simulink model "C02_PID_tuning_SISO"  (R2016b)
settings: Solver=ode45  StartTime=0.0  StopTime=4.5  RelTol=1e-3  EnableMultiTasking=on
model workspace (MAT data in the model file):
  sintez_sys_stab_optim : sldodialogs.data.SessionData (value not decoded)
undefined symbols (not defined in the file or in its folder): Kd, Ki, Kp
libraries: checkpacklib x1
settings Model: Creator=Gamno  LastModifiedBy=Maksim
settings DataIOCC: LimitDataPoints=on  SaveFormat=Array
settings OptimizationCC: ExpressionDepthLimit=2147483647  LifeSpan=inf
settings DebuggingCC: UnderspecifiedInitializationDetection=Classic  MergeDetectMultiDrivingBlocksExec=none  SolverPrmCheckMsg=warning  FcnCallInpInsideContextMsg=warning  StateNameClashWarn=warning  SFUnexpectedBacktrackingDiag=warning  SFNoUnconditionalDefaultTransitionDiag=warning  SFExecutionAtInitializationDiag=none
settings HardwareCC: ProdBitPerPointer=32  ProdBitPerSizeT=32  ProdBitPerPtrDiffT=32  ProdLargestAtomicFloat=None  ProdIntDivRoundTo=Undefined  ProdEndianess=Unspecified  ProdWordSize=32  ProdHWDeviceType=32-bit Generic
settings ModelReferenceCC: PropagateSignalLabelsOutOfModel=off
settings GRTTargetCC: TargetLangStandard=C89/C90 (ANSI)  GeneratePreprocessorConditionals=Disable all  CombineOutputUpdateFcns=off  GRTInterface=on
settings ConfigComp: CovMetricSettings=dw  CovHtmlReporting=on  CovSaveCumulativeToWorkspaceVar=on  CovSaveSingleToWorkspaceVar=on  CovExternalEMLEnable=off

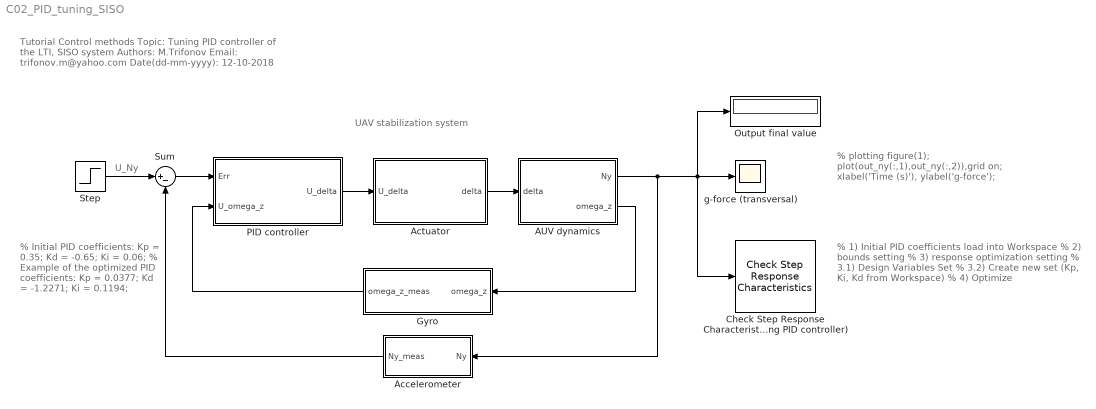
== system C02_PID_tuning_SISO ==
  note: UAV stabilization system
  note: % Initial PID coefficients:
      | Kp = 0.35;
      | Kd = -0.65;
      | Ki = 0.06;
      |
      | % Example of the optimized
      | PID coefficients:
      | Kp = 0.0377;
      | Kd = -1.2271;
      | Ki = 0.1194;
  note: U_Ny
  note: Tutorial Control methods
      | Topic: Tuning PID controller of the LTI, SISO system
      | Authors: M.Trifonov
      | Email: trifonov.m@yahoo.com
      | Date(dd-mm-yyyy): 12-10-2018
  note: % plotting
      | figure(1);
      | plot(out_ny(:,1),out_ny(:,2)),grid on;
      | xlabel('Time (s)'), ylabel('g-force');
  note: % 1) Initial PID coefficients load into Workspace
      | % 2) bounds setting
      | % 3) response optimization setting
      | % 3.1) Design Variables Set
      | % 3.2) Create new set (Kp, Ki, Kd from Workspace)
      | % 4) Optimize
  AUV dynamics : Subsystem
  Accelerometer : Subsystem
  Actuator : Subsystem
  Check Step Response Characteristics (tuning PID controller) : checkpacklib/Check Step Response  Characteristics  InstantiateOnLoad=on  enabled=on  stopWhenAssertionFail=off  export=off  ViewDlgPos=[1 41 1366 651]  OpenViewOnLoad=off  LaunchViewOnOpen=off  TimeUnits=seconds  EnableStepResponseBound=on  InitialValue=0  FinalValue=20  StepTime=0  RiseTime=1  PercentRise=90  SettlingTime=3  PercentSettling=1  PercentOvershoot=20  PercentUndershoot=1
  Gyro : Subsystem
  Output final value : Display
  PID controller : Subsystem
  Step : Step  Time=0  After=20  SampleTime=0
  Sum : Sum  Inputs=|+-
  g-force (transversal) : Scope
  wires:
  Step/1 -> Sum/1
  AUV dynamics/1(Ny) -> Output final value/1, Check Step Response Characteristics (tuning PID controller)/1, g-force (transversal)/1, Accelerometer/1(Ny)
  Sum/1 -> PID controller/1(Err)
  PID controller/1(U_delta) -> Actuator/1(U_delta)
  Actuator/1(delta) -> AUV dynamics/1(delta)
  AUV dynamics/2(omega_z) -> Gyro/1(omega_z)
  Gyro/1(omega_z_meas) -> PID controller/2(U_omega_z)
  Accelerometer/1(Ny_meas) -> Sum/2

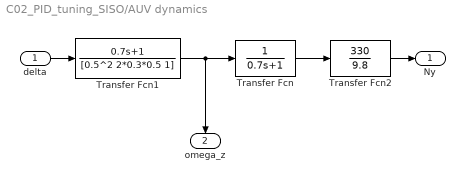
== system C02_PID_tuning_SISO/AUV dynamics ==
  delta : Inport
  Transfer Fcn : TransferFcn  Denominator=[0.7 1]
  Transfer Fcn1 : TransferFcn  Numerator=[0.7 1]  Denominator=[0.5^2 2*0.3*0.5 1]
  Transfer Fcn2 : TransferFcn  Numerator=[330]  Denominator=[9.8]
  Ny : Outport
  omega_z : Outport  Port=2
  wires:
  Transfer Fcn/1 -> Transfer Fcn2/1
  Transfer Fcn1/1 -> Transfer Fcn/1, omega_z/1
  delta/1 -> Transfer Fcn1/1
  Transfer Fcn2/1 -> Ny/1

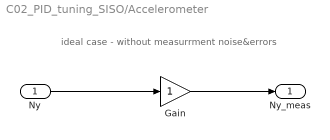
== system C02_PID_tuning_SISO/Accelerometer ==
  note: ideal case - without measurrment noise&errors
  Ny : Inport
  Gain : Gain
  Ny_meas : Outport
  wires:
  Gain/1 -> Ny_meas/1
  Ny/1 -> Gain/1

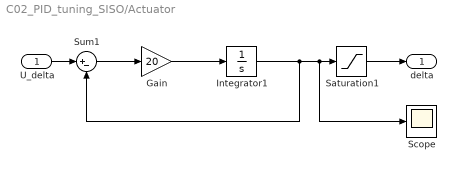
== system C02_PID_tuning_SISO/Actuator ==
  U_delta : Inport
  Gain : Gain  Gain=20
  Integrator1 : Integrator
  Saturation1 : Saturate  UpperLimit=30  LowerLimit=-30
  Scope : Scope
  Sum1 : Sum  Inputs=|+-
  delta : Outport
  wires:
  Sum1/1 -> Gain/1
  Integrator1/1 -> Sum1/2, Scope/1, Saturation1/1
  Gain/1 -> Integrator1/1
  U_delta/1 -> Sum1/1
  Saturation1/1 -> delta/1

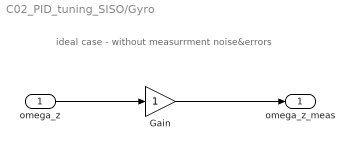
== system C02_PID_tuning_SISO/Gyro ==
  note: ideal case - without measurrment noise&errors
  omega_z : Inport
  Gain : Gain
  omega_z_meas : Outport
  wires:
  omega_z/1 -> Gain/1
  Gain/1 -> omega_z_meas/1

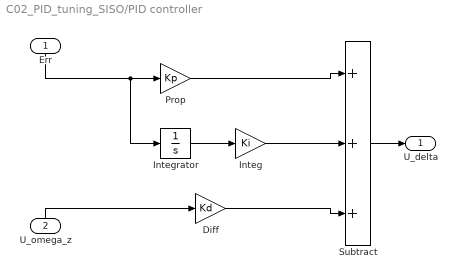
== system C02_PID_tuning_SISO/PID controller ==
  Err : Inport
  U_omega_z : Inport  Port=2
  Diff : Gain  Gain=Kd
  Integ : Gain  Gain=Ki
  Integrator : Integrator
  Prop : Gain  Gain=Kp
  Subtract : Sum  Inputs=+++
  U_delta : Outport
  wires:
  Integrator/1 -> Integ/1
  Integ/1 -> Subtract/2
  Prop/1 -> Subtract/1
  Err/1 -> Integrator/1, Prop/1
  Diff/1 -> Subtract/3
  U_omega_z/1 -> Diff/1
  Subtract/1 -> U_delta/1
